simulink model "untitled1"  (R2022b)
settings: Solver=VariableStepAuto  StartTime=0.0  StopTime=20  RelTol=1e-3
settings Model: Creator=Robert  LastModifiedBy=Robert

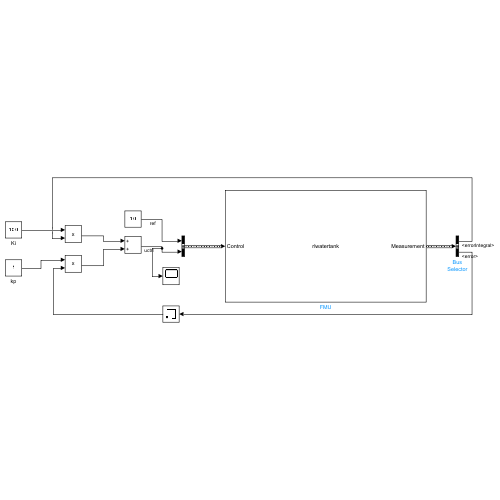
[thumbnail: Simulink's stored preview of the top-level diagram]
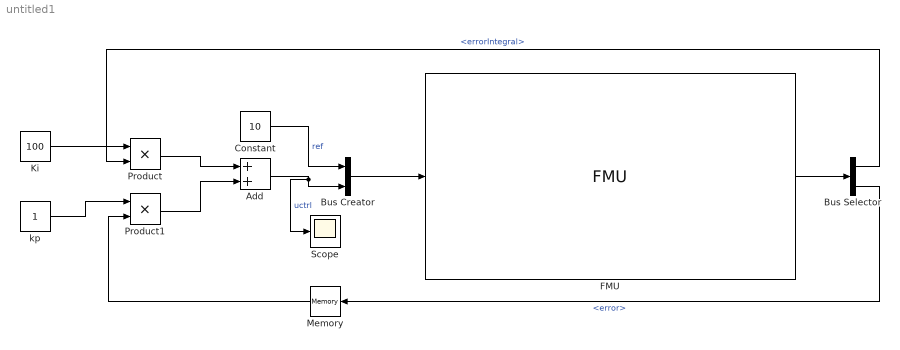
== system untitled1 ==
  Add : Sum
  Bus Creator : BusCreator  Inputs=2  OutDataTypeStr=Bus: Control  NonVirtualBus=on
  Bus Selector : BusSelector  OutputSignals=errorIntegral,error
  Constant : Constant  Value=10
  FMU : FMU  FMUName=rlwatertank.fmu  FMUMode=CoSimulation  FMUCreateBusObject=off
      mask Type: rlwatertank [Co-Simulation, v2.0]
      mask Display:
      | disp('rlwatertank');
      | port_label('output',1,'Measurement');
      | port_label('input',1,'Control');
  Ki : Constant  Value=100
  Memory : Memory
  Product : Product
  Product1 : Product
  Scope : Scope
  kp : Constant
  wires:
  Bus Creator/1 -> FMU/1
  FMU/1 -> Bus Selector/1
  Ki/1 -> Product/1
  Bus Selector/1 -> Product/2  "<errorIntegral>"
  kp/1 -> Product1/1
  Bus Selector/2 -> Memory/1  "<error>"
  Product1/1 -> Add/2
  Product/1 -> Add/1
  Constant/1 -> Bus Creator/1  "ref"
  Add/1 -> Scope/1, Bus Creator/2  "uctrl"
  Memory/1 -> Product1/2
